simulink model "Diesel_csi"  (R2017a)
settings: Solver=ode4  StartTime=0.0  StopTime=10.0  FixedStep=1e-6  MaxStep=1e-4  RelTol=1e-3
InitFcn:
  | SimulinkInit
values from neighbouring files (symbols this model uses):
  J = 0.3    [SimulinkInit.m]
  K1 = 1.15    [SimulinkInit.m]
  K2 = 1    [SimulinkInit.m]
  K3 = 1    [SimulinkInit.m]
  P = 0.1    [SimulinkInit.m]
  Tao1 = 0.5    [SimulinkInit.m]
  Tao2 = 0.125    [SimulinkInit.m]
undefined symbols (not defined in the file or in its folder): G, GF
libraries: powerlib x16, dsparch4 x3, powerlib_meascontrol x1, simulink x1
settings Model: Creator=Administrador  LastModifiedBy=Administrador
settings OptimizationCC: DefaultParameterBehavior=Inlined  PassReuseOutputArgsAs=Individual arguments
settings DebuggingCC: ParameterTunabilityLossMsg=error
settings SFSimCC: MATLABDynamicMemAlloc=off
settings RTWCC: SystemTargetFile=ert.tlc  TemplateMakefile=ert_default_tmf  Description=Embedded Coder  GenerateReport=on  IncludeHyperlinkInReport=on  LaunchReport=on  GenerateTraceInfo=on  GenerateTraceReport=on  GenerateTraceReportSl=on  GenerateTraceReportSf=on  GenerateTraceReportEml=on
settings CodeAppCC: ForceParamTrailComments=on  IgnoreCustomStorageClasses=off  OperatorAnnotations=on  SimulinkDataObjDesc=on  SFDataObjDesc=on  MATLABFcnDesc=on  InsertBlockDesc=on  MATLABSourceComments=on
settings ERTTargetCC: TargetLangStandard=C99 (ISO)  GenerateSampleERTMain=on  SupportContinuousTime=on  SupportNonInlinedSFcns=on  SupportVariableSizeSignals=on  InlinedParameterPlacement=NonHierarchical  ERTCustomFileTemplate=example_file_process.tlc

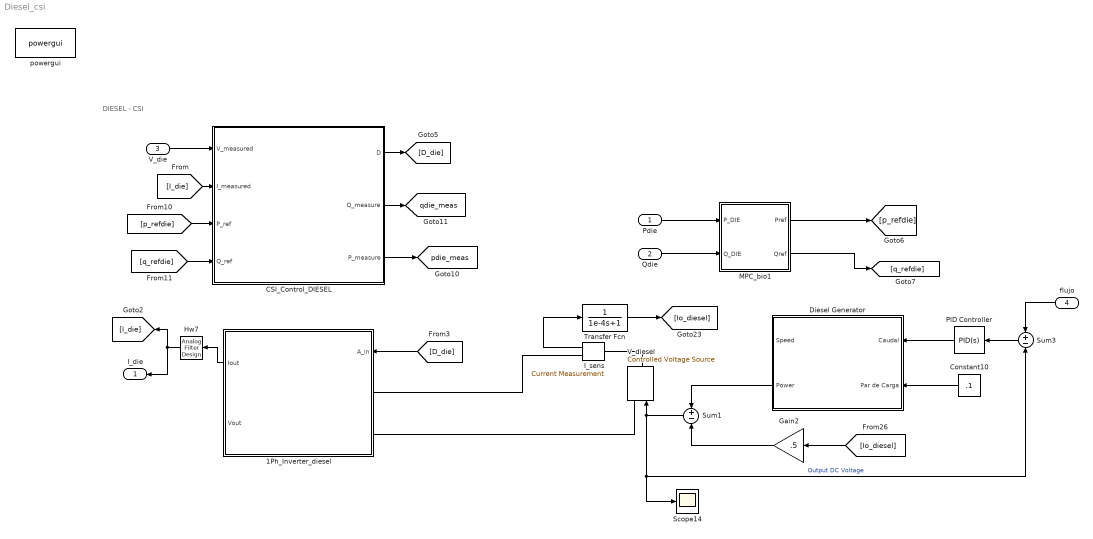
== system Diesel_csi ==
  note: DIESEL - CSI
  Pdie : Inport  PortDimensions=1
  Qdie : Inport  Port=2  PortDimensions=1
  V_die : Inport  Port=3
  flujo : Inport  Port=4
  1Ph_Inverter_diesel : Subsystem  mask{st_time=0, f_sw=12000, samp_f=1e-6}
      mask prompts: st_time "Tiempo muerto (Start)"; f_sw "Switching frequency"; samp_f "Sampling frequency"
      mask Display:
      | port_label('input', 1, 'd', 'texmode', 'on')
      | 
      | port_label('lconn', 1, 'DC +')
      | port_label('lconn', 2, 'DC -')
      | 
      | 
      | port_label('rconn', 1, 'V_{out+}')
      | port_label('rconn', 2, 'B_{out-}')
      | 
      | 
      | port_label('output', 1, 'I_{out}', 'texmode', 'on')
      | port_label('output', 2, 'V_{out}', 'texmode', 'on')
      | 
      | plot([0.1 .9], [0.1 .9])
      | plot([0.2 .4], [.7 .7])
      | plot([0.2 .24], [.65 .65])
      | plot([0.28 .32], [.65 .65])
      | plot([0.36 .40], [.65 .65])
      | 
      | plot([.5:.01:.7], .25+sin(30*[.2:.01:.4])/10)
  CSI_Control_DIESEL : Subsystem  mask{A=[0.0201   -0.039932     0.01986], B=[1     -1.9966       0.998], T=0.0001, st_time=.3, Dn=[1     -1.0364], Dd=[1    -0.96364]}
      mask prompts: A "Numerador del control PR(z)"; B "Denominador del control PR(z)"; T "Tiempo de muestreo"; st_time "Tiempo_muerto"; Dn "Dn (Numerador de D(z))"; Dd "Dd (numerador de D(z))"
      mask DialogControl descripcion Prompt: Lazo de control de corriente para inversor monofasico. La entrada es un setpoint de potencia [P, Q]. Con ese setpoint se calcula la referencia de corriente sinusoidal deacuerdo a la tension medida de la red. Por lo anterior este controlador solo es valido para un inversor conectado a la red pues hara que se comporte como un CSI.
      mask DialogControl Control2 Prompt: Dn y Dd corresponden al numerador y denominador de la funcion de transferencia en Z (denominada D(z)) que hara un desfase de 90 de las señales medidas de tension y corriente del inversor. Estos desfases permiten mimificar las señales alfa y beta, de esta forma usar la misma teoria de potencia instantanea para el caso monofasico.
  Constant10 : Constant  Value=.1
  Diesel Generator : Subsystem
  Gain2 : Gain  Gain=.5
  Hw7 : dsparch4/Analog Filter Design  method=Bessel  filttype=Lowpass  N=2  Wlo=7000*2*pi  Whi=80  Rp=2  Rs=80
  I_sens : powerlib/Measurements/Current Measurement  PhasorSimulation=off  OutputType=Complex  PSBequivalent=0
  MPC_bio1 : Subsystem
  PID Controller : simulink/Continuous/PID Controller  Controller=PID  TimeDomain=Continuous-time  SampleTime=-1  IntegratorMethod=Forward Euler  FilterMethod=Forward Euler  Form=Parallel  UseFilter=on  ControllerParametersSource=internal  P=0.000853612192208084  I=3.94394231511782e-05  D=0.00224356290205903  N=0.155980576752107  InitialConditionSource=internal  InitialConditionForIntegrator=0  InitialConditionForFilter=0  ExternalReset=none  LimitOutput=off  UpperSaturationLimit=inf  LowerSaturationLimit=-inf  LinearizeAsGain=on  AntiWindupMode=none  Kb=1  TrackingMode=off  Kt=1  PParamMin=[]  PParamMax=[]  IParamMin=[]  IParamMax=[]  DParamMin=[]  DParamMax=[]  NParamMin=[]  NParamMax=[]  KbParamMin=[]  KbParamMax=[]  KtParamMin=[]  KtParamMax=[]  POutMin=[]  POutMax=[]  IOutMin=[]  IOutMax=[]  DOutMin=[]  DOutMax=[]  NOutMin=[]  NOutMax=[]  KbOutMin=[]  KbOutMax=[]  KtOutMin=[]  KtOutMax=[]  IntegratorOutMin=[]  IntegratorOutMax=[]  FilterOutMin=[]  FilterOutMax=[]  SumOutMin=[]  SumOutMax=[]  SumI1OutMin=[]  SumI1OutMax=[]  SumI2OutMin=[]  SumI2OutMax=[]  SumI3OutMin=[]  SumI3OutMax=[]  SumDOutMin=[]  SumDOutMax=[]  SaturationOutMin=[]  SaturationOutMax=[]  IntegratorContinuousStateAttributes=''  IntegratorStateMustResolveToSignalObject=off  IntegratorRTWStateStorageClass=Auto  FilterContinuousStateAttributes=''  FilterStateMustResolveToSignalObject=off  FilterRTWStateStorageClass=Auto  DifferentiatorICPrevScaledInput=0  DifferentiatorOutMin=[]  DifferentiatorOutMax=[]  InitialConditionSetting=State (most efficient)
  Scope14 : Scope
  Sum1 : Sum  Inputs=+-
  Sum3 : Sum  Inputs=+-
  Transfer Fcn : TransferFcn  Denominator=[1e-4 1]
  V_diesel : powerlib/Electrical Sources/Controlled Voltage Source  Initialize=on  Source_Type=AC  Amplitude=0  Phase=0  Frequency=0  Measurements=None
  powergui : powerlib/powergui  Priority=1  SimulationMode=Discrete  SampleTime=1e-6  frequency=60  Iterations=50  frequencyindice=0  Pbase=100e6  ErrMax=1e-4  UnitsV=kV  UnitsW=MW  buscounter=0  FunctionMessages=off  echomessages=off  EnableUseOfTLC=off  CurrentSourceSwitches=off  DisableSnubberDevices=off  DisableRonSwitches=off  DisableVfSwitches=off  DisplayEquations=off  SolverType=Tustin/Backward Euler (TBE)  Interpol=off  ExternalGateDelay=off  methode=off  Ts=100  x0status=blocks  SPID=on  SwTol=0  HookPort=off  RestoreLinks=warning  ResistiveCurrentMeasurement=off  Frange=[0:2:500]  Ylog=off  Xlog=on  ShowGrid=off  save=off  variable=ZData  structure=0  ZoomFFT=off  StartTime=0.0  cycles=1  DisplayStyle=1  fundamental=60  FreqAxis=off  MaxFrequency=1000  frequencyindicesteady=1  RmsSteady=1  display=off
  I_die : Outport
  tag scope: pdie_meas=global, qdie_meas=global
  wires:
  [p_refdie] -> CSI_Control_DIESEL/3(P_ref)
  [I_die] -> CSI_Control_DIESEL/2(I_measured)
  CSI_Control_DIESEL/1(D) -> [D_die]
  [D_die] -> 1Ph_Inverter_diesel/1(A_in)
  CSI_Control_DIESEL/2(Q_measure) -> [qdie_meas]
  MPC_bio1/2(Qref) -> [q_refdie]
  Pdie/1 -> MPC_bio1/1(P_DIE)
  1Ph_Inverter_diesel/1(Iout) -> Hw7/1
  Hw7/1 -> I_die/1, [I_die]
  Qdie/1 -> MPC_bio1/2(Q_DIE)
  I_sens/1 -> Transfer Fcn/1
  PID Controller/1 -> Diesel Generator/1(Caudal)
  flujo/1 -> Sum3/1
  Transfer Fcn/1 -> [Io_diesel]
  [Io_diesel] -> Gain2/1
  V_die/1 -> CSI_Control_DIESEL/1(V_measured)
  CSI_Control_DIESEL/3(P_measure) -> [pdie_meas]
  Sum3/1 -> PID Controller/1
  Sum1/1 -> Scope14/1, Sum3/2, V_diesel/1  "Output DC Voltage"
  Constant10/1 -> Diesel Generator/2(Par de Carga)
  MPC_bio1/1(Pref) -> [p_refdie]
  Diesel Generator/2(Power) -> Sum1/1
  Gain2/1 -> Sum1/2
  [q_refdie] -> CSI_Control_DIESEL/4(Q_ref)
  connections:
  I_sens/LConn1 -- V_diesel/RConn1
  I_sens/RConn1 -- 1Ph_Inverter_diesel/LConn1
  V_diesel/LConn1 -- 1Ph_Inverter_diesel/LConn2

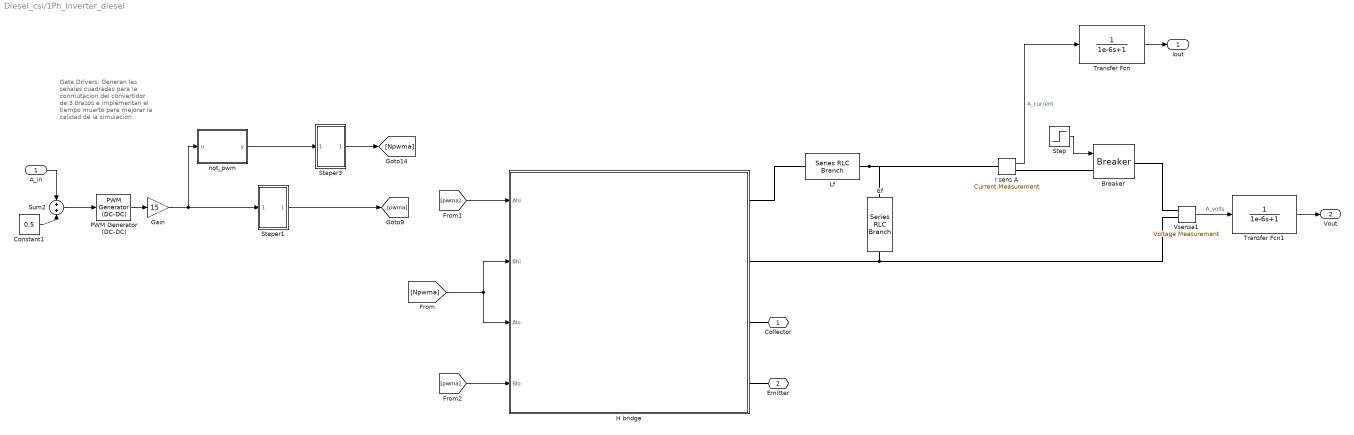
== system Diesel_csi/1Ph_Inverter_diesel ==
  note: Gate Drivers: Generan las señales cuadradas para
      | la conmutacion del convertidor de 3 brazos e implementan el
      | tiempo muerto para mejorar la calidad de la simulacion
  A_in : Inport
  Breaker : powerlib/Elements/Breaker  InitialState=0  SwitchingTimes="[1/60  5/60]"  External=on  BreakerResistance=0.01  SnubberResistance=1e6  SnubberCapacitance=inf  Measurements=None  MoreParameters=on  NoBreakLoop=off
      settings: SourceProductName=Simscape Power Systems
  Cf : powerlib/Elements/Series RLC Branch  LConnTagsString=__new0  RConnTagsString=__new0  BranchType=C  Resistance=1  Inductance=1e-3  SetiL0=off  InitialCurrent=0  Capacitance=22e-6  Setx0=off  InitialVoltage=0  Measurements=None
  Constant1 : Constant  Value=0.5
  Gain : Gain  Gain=15
  H bridge : Subsystem
      mask Display:
      | port_label('input', 1, '\fontsize{12} Ahi', 'texmode', 'on')
      | port_label('input', 2, '\fontsize{12} Alo', 'texmode', 'on')
      | port_label('input', 3, '\fontsize{12} Bhi', 'texmode', 'on')
      | port_label('input', 4, '\fontsize{12} Blo', 'texmode', 'on')
      | 
      | 
      | port_label('rconn', 1, '\fontsize{12} V_{out} +', 'texmode', 'on')
      | port_label('rconn', 2, '\fontsize{12} V_{out} -', 'texmode', 'on')
      | 
      | port_label('rconn', 3, '\fontsize{12} Collector', 'texmode', 'on')
      | port_label('rconn', 4, '\fontsize{12} Emitter', 'texmode', 'on')
      | 
      | lvx = [.1 .1];
      | lvy = [.1 .2];
      | lhx = [.1 .2];
      | lhy = [.1 .1];
      | 
      | 
      | % se dibujan los interruptores de la izquierda
      | plot(lvx+.07, lvy*.8+.028+.1)
      | plot(lvx+.1, lvy+.1)
      | plot(lhx*.5+.15, lhy+.1)
      | plot(lhx*.5+.15, lhy+.2)
      | plot(lhx*.5+.07, lhy+.15)
      | 
      | d=0.5;
      | 
      | plot(lvx+.07, lvy*.8+.028+.1+d)
      | plot(lvx+.1, lvy+.1+d)
      | plot(lhx*.5+.15, lhy+.1+d)
      | plot(lhx*.5+.15, lhy+.2+d)
      | plot(lhx*.5+.07, lhy+.15+d)
      | 
      | 
      | % se dibujan los interruptores del medio
      | h=.3;
      | 
      | %plot(lvx+.07+h, lvy*.8+.028+.1)
      | %plot(lvx+.1+h, lvy+.1)
      | %plot(lhx*.5+.15+h, lhy+.1)
      | %plot(lhx*.5+.15+h, lhy+.2)
      | %plot(lhx*.5+.07+h, lhy+.15)
      | 
      | %plot(lvx+.07+h, lvy*.8+.028+.1+d)
      | %plot(lvx+.1+h, lvy+.1+d)
      | %plot(lhx*.5+.15+h, lhy+.1+d)
      | %plot(lhx*.5+.15+h, lhy+.2+d)
      | %plot(lhx*.5+.07+h, lhy+.15+d)
      | 
      | % se dibujan los interruptores de la derecha
      | h=.6
      | 
      | plot(lvx+.07+h, lvy*.8+.028+.1)
      | plot(lvx+.1+h, lvy+.1)
      | plot(lhx*.5+.15+h, lhy+.1)
      | plot(lhx*.5+.15+h, lhy+.2)
      | plot(lhx*.5+.07+h, lhy+.15)
      | 
      | plot(lvx+.07+h, lvy*.8+.028+.1+d)
      | plot(lvx+.1+h, lvy+.1+d)
      | plot(lhx*.5+.15+h, lhy+.1+d)
      | plot(lhx*.5+.15+h, lhy+.2+d)
      | plot(lhx*.5+.07+h, lhy+.15+d)
      | 
      | 
      | % se conectan los interruptores.
      | plot(lvx+.15, lvy*4-.1)
      | %plot(lvx+.15+.3, lvy*4-.1)
      | plot(lvx+.15+.6, lvy*4-.1)
      | 
      | 
      | plot(lvx+.15, lvy+.7)
      | %plot(lvx+.15+.3, lvy+.7)
      | plot(lvx+.15+.6, lvy+.7)
      | 
      | plot(lvx+.15, lvy)
      | %plot(lvx+.15+.3, lvy)
      | plot(lvx+.15+.6, lvy)
      | 
      | plot(lhx*6-.35, lhy)
      | plot(lhx*6-.35, lhy+.8)
      | 
      | % raul esteban alzate 313 515 86 11
  I sens A : powerlib/Measurements/Current Measurement  PhasorSimulation=off  OutputType=Complex  PSBequivalent=0
  Lf : powerlib/Elements/Series RLC Branch  LConnTagsString=__new0  RConnTagsString=__new0  BranchType=RL  Resistance=.1  Inductance=30e-3  SetiL0=off  InitialCurrent=0  Capacitance=1e-6  Setx0=off  InitialVoltage=0  Measurements=None
  PWM Generator (DC-DC) : powerlib_meascontrol/Pulse & Signal Generators/PWM Generator (DC-DC)  Fsw=f_sw  Ts=samp_f
  Step : Step  Time=st_time  SampleTime=0
  Steper1 : Subsystem
  Steper3 : Subsystem
  Sum2 : Sum
  Transfer Fcn : TransferFcn  Denominator=[1e-6 1]
  Transfer Fcn1 : TransferFcn  Denominator=[1e-6 1]
  Vsensa1 : powerlib/Measurements/Voltage Measurement  PhasorSimulation=off  OutputType=Complex  PSBequivalent=0
  not_pwm : MATLAB Function  TreatAsAtomicUnit=on
  Collector : PMIOPort  Port=1  Side=Left
  Emitter : PMIOPort  Port=2  Side=Left
  Iout : Outport
  Vout : Outport  Port=2
  wires:
  Vsensa1/1 -> Transfer Fcn1/1  "A_volts"
  I sens A/1 -> Transfer Fcn/1  "A_current"
  [pwma] -> H bridge/4(Blo)
  [Npwma] -> H bridge/3(Alo), H bridge/2(Bhi)
  [pwma] -> H bridge/1(Ahi)
  Gain/1 -> not_pwm/1(u), Steper1/1(In1)
  Steper3/1(Out1) -> [Npwma]
  Steper1/1(Out1) -> [pwma]
  A_in/1 -> Sum2/1
  Constant1/1 -> Sum2/2
  PWM Generator (DC-DC)/1 -> Gain/1
  Sum2/1 -> PWM Generator (DC-DC)/1
  not_pwm/1(y) -> Steper3/1(In1)
  Transfer Fcn/1 -> Iout/1
  Transfer Fcn1/1 -> Vout/1
  Step/1 -> Breaker/1
  connections:
  Cf/RConn1 -- Vsensa1/LConn2 -- H bridge/RConn2
  Lf/LConn1 -- H bridge/RConn1
  H bridge/RConn4 -- Emitter/RConn1
  H bridge/RConn3 -- Collector/RConn1
  Breaker/LConn1 -- I sens A/RConn1
  Vsensa1/LConn1 -- Breaker/RConn1
  Lf/RConn1 -- I sens A/LConn1 -- Cf/LConn1

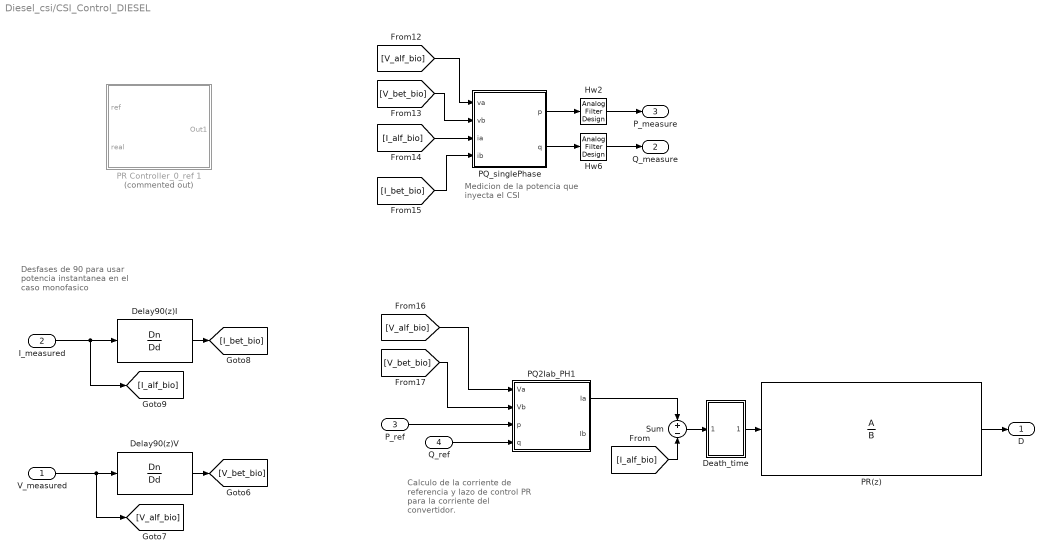
== system Diesel_csi/CSI_Control_DIESEL ==
  note: Calculo de la corriente de referencia
      | y lazo de control PR para la corriente
      | del convertidor.
  note: Desfases de 90 para usar potencia
      | instantanea en el caso monofasico
  note: Medicion de la potencia que inyecta el CSI
  V_measured : Inport
  I_measured : Inport  Port=2
  P_ref : Inport  Port=3
  Q_ref : Inport  Port=4
  Death_time : Subsystem
  Delay90(z)I : DiscreteTransferFcn  Numerator=Dn  Denominator=Dd  SampleTime=T
  Delay90(z)V : DiscreteTransferFcn  Numerator=Dn  Denominator=Dd  SampleTime=T
  Hw2 : dsparch4/Analog Filter Design  method=Bessel  filttype=Lowpass  N=4  Wlo=30*2*pi  Whi=80  Rp=2  Rs=80
  Hw6 : dsparch4/Analog Filter Design  method=Bessel  filttype=Lowpass  N=4  Wlo=30*2*pi  Whi=80  Rp=2  Rs=80
  PQ2Iab_PH1 : MATLAB Function  TreatAsAtomicUnit=on
  PQ_singlePhase : MATLAB Function  TreatAsAtomicUnit=on
  PR Controller_0_ref 1 : Subsystem  Commented=on  mask{Kp=40/100, Ki=200, wa=2, w0=60*2*pi, st_time=1e-3}
      mask prompts: Kp "Ganancia Proporcional"; Ki "Ganancia Integral"; wa "Ancho camapana resonancia"; w0 "Frecuencia Central"; st_time "Tiempo muerto (Start)"
      mask Display:
      | port_label('input',1,'ref')
      | port_label('input',2,'sens')
      | port_label('output',1,'out')
      | 
      | plot(.4+[0:.01:pi/10], .32+sin(40*[0:.01:pi/10])/13)
      | 
      | plot([.4 .6],.05+[.5 .7])
      | plot([.4 .6],.05+[.9 .7])
      | plot([.4 .4],.05+[.9 .5])
      | 
      | text(.27,.37,'\fontsize{25} \int', 'texmode', 'on')
  PR(z) : DiscreteTransferFcn  Numerator=A  Denominator=B  SampleTime=T
  Sum : Sum  Inputs=+-
  D : Outport
  Q_measure : Outport  Port=2
  P_measure : Outport  Port=3
  wires:
  PR(z)/1 -> D/1
  Sum/1 -> Death_time/1(In1)
  PQ2Iab_PH1/1(Ia) -> Sum/1
  [I_alf_bio] -> Sum/2
  Death_time/1(Out1) -> PR(z)/1
  Q_ref/1 -> PQ2Iab_PH1/4(q)
  P_ref/1 -> PQ2Iab_PH1/3(p)
  PQ_singlePhase/2(q) -> Hw6/1
  V_measured/1 -> [V_alf_bio], Delay90(z)V/1
  [V_alf_bio] -> PQ_singlePhase/1(va)
  [V_bet_bio] -> PQ_singlePhase/2(vb)
  Delay90(z)V/1 -> [V_bet_bio]
  Hw2/1 -> P_measure/1
  [V_alf_bio] -> PQ2Iab_PH1/1(Va)
  [I_alf_bio] -> PQ_singlePhase/3(ia)
  [I_bet_bio] -> PQ_singlePhase/4(ib)
  Delay90(z)I/1 -> [I_bet_bio]
  [V_bet_bio] -> PQ2Iab_PH1/2(Vb)
  Hw6/1 -> Q_measure/1
  PQ_singlePhase/1(p) -> Hw2/1
  I_measured/1 -> [I_alf_bio], Delay90(z)I/1

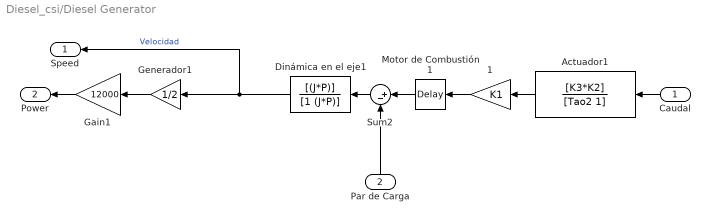
== system Diesel_csi/Diesel Generator ==
  Caudal : Inport
  Par de Carga : Inport  Port=2
  " 1" : Gain  Gain=K1
  " Generador1" : Gain  Gain=1/2
  Actuador1 : TransferFcn  Numerator=[K3*K2]  Denominator=[Tao2 1]
  Dinámica en el eje1 : TransferFcn  Numerator=[(J*P)]  Denominator=[1 (J*P)]
  Gain1 : Gain  Gain=12000
  Motor de Combustión1 : TransportDelay  DelayTime=Tao1
  Sum2 : Sum  Inputs=|+-
  Speed : Outport
  Power : Outport  Port=2
  wires:
  " 1"/1 -> Motor de Combustión1/1
  " Generador1"/1 -> Gain1/1
  Motor de Combustión1/1 -> Sum2/1
  Actuador1/1 -> " 1"/1
  Dinámica en el eje1/1 -> Speed/1, " Generador1"/1  "Velocidad"
  Sum2/1 -> Dinámica en el eje1/1
  Caudal/1 -> Actuador1/1
  Par de Carga/1 -> Sum2/2
  Gain1/1 -> Power/1

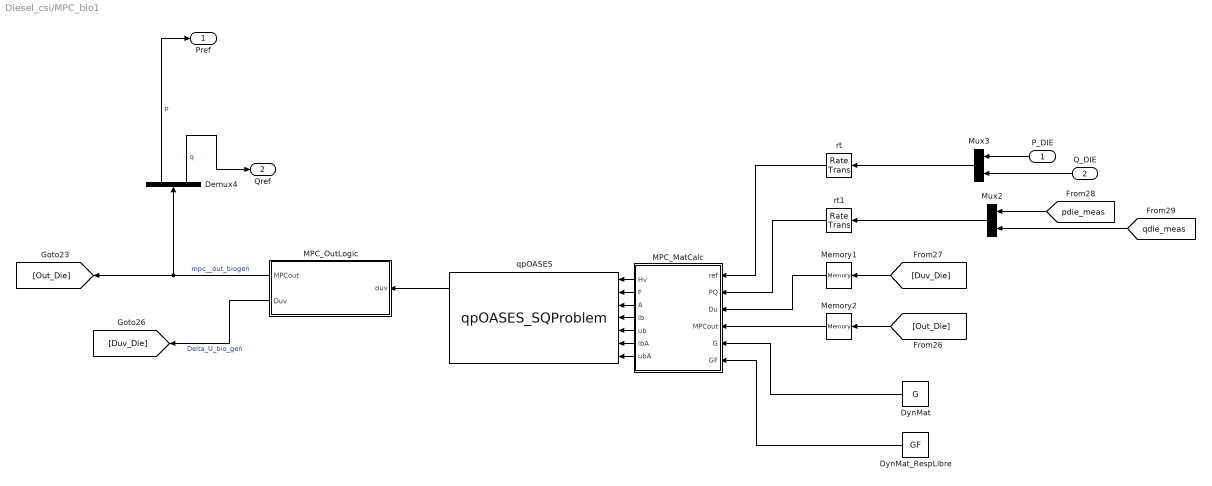
== system Diesel_csi/MPC_bio1 ==
  P_DIE : Inport
  Q_DIE : Inport  Port=2
  Demux4 : Demux  Outputs=2
  DynMat : Constant  Value=G
  DynMat_RespLibre : Constant  Value=GF
  MPC_MatCalc : MATLAB Function  TreatAsAtomicUnit=on  SystemSampleTime=1e-3
      settings: MinAlgLoopOccurrences=on
  MPC_OutLogic : MATLAB Function  TreatAsAtomicUnit=on
      settings: MinAlgLoopOccurrences=on
  Memory1 : Memory
  Memory2 : Memory
  Mux2 : Mux  Inputs=2
  Mux3 : Mux  Inputs=2
  qpOASES : S-Function  FunctionName=qpOASES_SQProblem  SFunctionDeploymentMode=off  EnableBusSupport=off
  rt : RateTransition  X0=[0 0]  OutPortSampleTime=1e-3
  rt1 : RateTransition  X0=[0 0]  OutPortSampleTime=1e-3
  Pref : Outport
  Qref : Outport  Port=2
  wires:
  [Out_Die] -> Memory2/1
  MPC_MatCalc/7(ubA) -> qpOASES/7
  MPC_MatCalc/6(lbA) -> qpOASES/6
  MPC_MatCalc/2(F) -> qpOASES/2
  rt1/1 -> MPC_MatCalc/2(PQ)
  Memory1/1 -> MPC_MatCalc/3(Du)
  [Duv_Die] -> Memory1/1
  MPC_MatCalc/5(ub) -> qpOASES/5
  MPC_OutLogic/1(MPCout) -> [Out_Die], Demux4/1  "mpc__out_biogen"
  DynMat_RespLibre/1 -> MPC_MatCalc/6(GF)
  DynMat/1 -> MPC_MatCalc/5(G)
  Demux4/1 -> Pref/1  "p"
  Memory2/1 -> MPC_MatCalc/4(MPCout)
  MPC_MatCalc/3(A) -> qpOASES/3
  MPC_MatCalc/1(Hv) -> qpOASES/1
  MPC_OutLogic/2(Duv) -> [Duv_Die]  "Delta_U_bio_gen"
  MPC_MatCalc/4(lb) -> qpOASES/4
  rt/1 -> MPC_MatCalc/1(ref)
  qpOASES/1 -> MPC_OutLogic/1(duv)
  Mux2/1 -> rt1/1
  Mux3/1 -> rt/1
  [pdie_meas] -> Mux2/1
  Q_DIE/1 -> Mux3/2
  [qdie_meas] -> Mux2/2
  Demux4/2 -> Qref/1  "q"
  P_DIE/1 -> Mux3/1

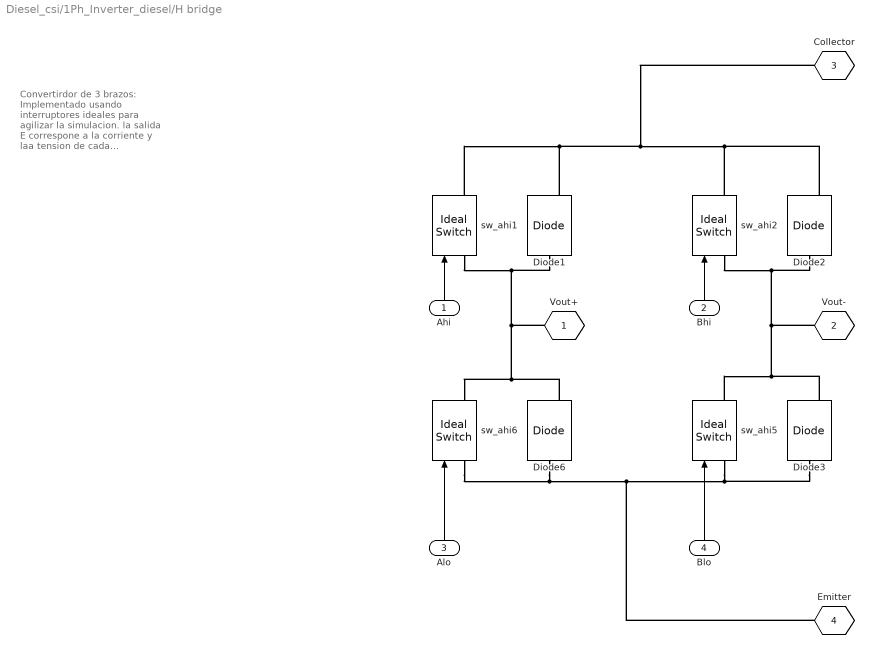
== system Diesel_csi/1Ph_Inverter_diesel/H bridge ==
  note: Convertirdor de 3 brazos:
      |
      | Implementado usando interruptores
      | ideales para agilizar la simulacion.
      | la salida E correspone a la corriente y laa
      | tension de cada componente
      | (sea interruptor o diodo) y su respectiva
      | corriente. no tienen puerto de salida ya que no
      | son relevantes para lo que se desea simular.
      |
      | si g=0 interruptor no conduce.
      | si g=1 interruptor conduce.
      |
      | conmutacion ocurre instantaneamente sin
      | retardo.
  Ahi : Inport
  Bhi : Inport  Port=2
  Alo : Inport  Port=3
  Blo : Inport  Port=4
   sw_ahi{1..2,5..6} (4 alike) : powerlib/Power Electronics/Ideal Switch  Ron=0.1  Lon=0  IC=0  Rs=1e6  Cs=10e-12  Measurements=on
  Diode{1..3,6} (4 alike) : powerlib/Power Electronics/Diode  Ron=.2  Lon=0  Vf=0.8  IC=0  UseSnubber=0  Rs=0  Cs=0  Measurements=on
  " Vout+" : PMIOPort  Tag=PMCPort  Port=1  Side=Right
  Vout- : PMIOPort  Tag=PMCPort  Port=2  Side=Right
  Collector : PMIOPort  Tag=PMCPort  Port=3  Side=Right
  Emitter : PMIOPort  Tag=PMCPort  Port=4  Side=Right
  wires:
  Bhi/1 -> " sw_ahi2"/1
  Blo/1 -> " sw_ahi5"/1
  Ahi/1 -> " sw_ahi1"/1
  Alo/1 -> " sw_ahi6"/1
  connections:
  " sw_ahi1"/LConn1 -- Diode1/LConn1 -- " Vout+"/RConn1 -- Diode6/RConn1 -- " sw_ahi6"/RConn1
  " sw_ahi2"/RConn1 -- Diode1/RConn1 -- " sw_ahi1"/RConn1 -- Collector/RConn1 -- Diode2/RConn1
  " sw_ahi5"/LConn1 -- " sw_ahi6"/LConn1 -- Diode6/LConn1 -- Emitter/RConn1 -- Diode3/LConn1
  " sw_ahi5"/RConn1 -- Diode2/LConn1 -- " sw_ahi2"/LConn1 -- Vout-/RConn1 -- Diode3/RConn1

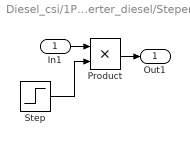
== system Diesel_csi/1Ph_Inverter_diesel/Steper1 ==
  In1 : Inport
  Product : Product
  Step : Step  Time=st_time  SampleTime=samp_f
  Out1 : Outport
  wires:
  Product/1 -> Out1/1
  In1/1 -> Product/1
  Step/1 -> Product/2

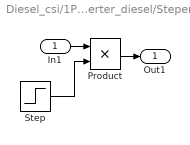
== system Diesel_csi/1Ph_Inverter_diesel/Steper3 ==
  In1 : Inport
  Product : Product
  Step : Step  Time=st_time  SampleTime=samp_f
  Out1 : Outport
  wires:
  Step/1 -> Product/2
  In1/1 -> Product/1
  Product/1 -> Out1/1

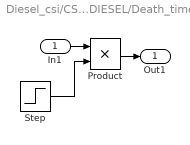
== system Diesel_csi/CSI_Control_DIESEL/Death_time ==
  In1 : Inport
  Product : Product
  Step : Step  Time=st_time  SampleTime=T
  Out1 : Outport
  wires:
  Step/1 -> Product/2
  In1/1 -> Product/1
  Product/1 -> Out1/1

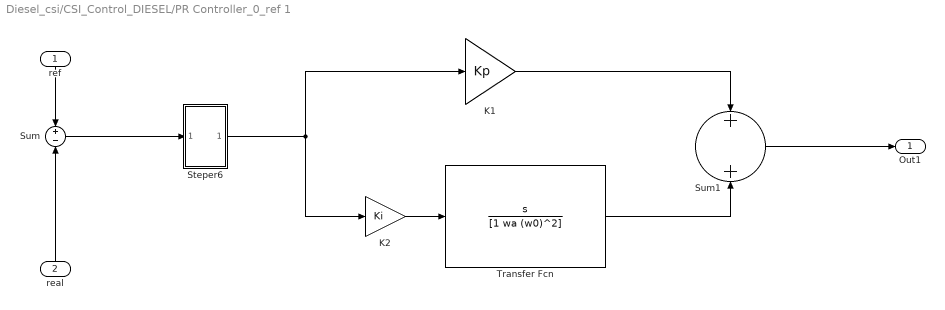
== system Diesel_csi/CSI_Control_DIESEL/PR Controller_0_ref 1 ==
  ref : Inport
  real : Inport  Port=2
  K1 : Gain  Gain=Kp
  K2 : Gain  Gain=Ki
  Steper6 : Subsystem
  Sum : Sum  Inputs=+-
  Sum1 : Sum  Inputs=+|+
  Transfer Fcn : TransferFcn  Numerator=[1 0]  Denominator=[1 wa (w0)^2]
  Out1 : Outport
  wires:
  Sum1/1 -> Out1/1
  Steper6/1(Out1) -> K2/1, K1/1
  K2/1 -> Transfer Fcn/1
  Transfer Fcn/1 -> Sum1/2
  K1/1 -> Sum1/1
  Sum/1 -> Steper6/1(In1)
  ref/1 -> Sum/1
  real/1 -> Sum/2

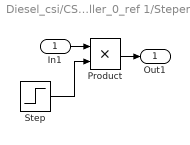
== system Diesel_csi/CSI_Control_DIESEL/PR Controller_0_ref 1/Steper6 ==
  In1 : Inport
  Product : Product
  Step : Step  Time=st_time  SampleTime=0
  Out1 : Outport
  wires:
  Step/1 -> Product/2
  In1/1 -> Product/1
  Product/1 -> Out1/1

== matlab function Diesel_csi/1Ph_Inverter_diesel/not_pwm ==
  data: u input; y output
function y = fcn(u)
%#codegen

if(u==0 || u<0)
    a=15;
else
    a=0;
end;

y = a;

== matlab function Diesel_csi/CSI_Control_DIESEL/PQ2Iab_PH1 ==
  data: Va input; Ia output; Vb input; p input; q input; Ib output
function [Ia, Ib] = fcn(Va, Vb, p, q)
%#codegen

% divide by zero protection
if(abs((Va^2+Vb^2))<=1000*eps(0))
    det = 1/eps(0);
else
    det = 1/(Va^2+Vb^2); % constante auxiliar
end;
%det = 1/(Va^2+Vb^2);

Mat = det*[Va Vb; Vb -Va];
Iab = Mat*[2*p;2*q];

Iaaux = Iab(1);
Ibaux = Iab(2);

ilim=1e3;

if(Iaaux>ilim)
    Iaaux=ilim;
end;
if(Iaaux<-ilim)
    Iaaux =-ilim;    
end;

if(isnan(Iaaux))
    Iaaux=0;
end;
%-----------------


if(Ibaux>ilim)
    Ibaux=ilim;
end;
if(Ibaux<-ilim)
    Ibaux =-ilim;    
end;

if(isnan(Ibaux))
    Ibaux=0;
end;
%-----------------


Ia = Iaaux;
Ib = Ibaux;

== matlab function Diesel_csi/CSI_Control_DIESEL/PQ_singlePhase ==
  data: va input; p output; vb input; ia input; ib input; q output
function [p, q] = fcn(va, vb, ia, ib)
% Esta funcion calcula la potencia activa y reactiva instantanea
% para el caso mnosofasico. En la revision de 2 papers he observado
% que una manera de extender la teoria de potencia al caso monofasico
% es asumiendo la tension o corriente de una fase como la componente
% alpha y hacer un desfase de 90 grados para obtener una version
% artificial de beta.

paux=va*ia+vb*ib;
if(paux > 20e4)
    paux = 20e4;
end
if(paux < -20e4)
    paux = -20e-4;
end

p = paux/2; % potencia activa instantanea

qaux = vb*ia-va*ib;

if(qaux>20e4)
    qaux=20e4;
end
if(qaux<-20e4)
    qaux=-20e4;
end

q = qaux/2; % potencia reactiva instantanea

== matlab function Diesel_csi/MPC_bio1/MPC_MatCalc ==
  data: ref input; PQ input; Hv output; F output; A output; lb output; ub output; lbA output; ubA output; Du input; MPCout input; G input; GF input
function [Hv, F, A, lb, ub, lbA, ubA] = MPC(ref, PQ, Du, MPCout, G, GF)

%%parametros del MPC


p = 100; % horizonte de prediccion
Nu = 100; % horizonte de control


%% Calculo de la salida de control.

H = G'*G+eye(2*Nu)*3000; % parte cuadratica del qp

ym = [ ones(p, 1)*PQ(1); ones(p, 1)*PQ(2) ]; % vector de la medida de tempearatura actual.

w = [ ones(p, 1)*ref(1); ones(p, 1)*ref(2) ]; % vector señal setpoint.

L = GF*Du+ym; % respuesta libre.

F = 2*(L-w)'*G; % parte lineal del problema qp.

A = zeros(1, 4*Nu*Nu);

lbA = zeros(1, 2*Nu);

ubA = zeros(1, 2*Nu);

Hv = M2V(H);

hip = HiBound(MPCout(1), 600, 10);
hiq = HiBound(MPCout(2), 5000, 1000);

lop = LowBound(MPCout(1), -100, -10);
loq = LowBound(MPCout(2), -100, -1000);

lb = [ones(1, Nu)*lop ones(1, Nu)*loq];
ub = [ones(1, Nu)*hip ones(1, Nu)*hiq];
end

% el control mpc implementado halla mediante programacion cuadratica
% los delta de u optimos deacuerdo a la funcion de coste. por este motivo
% es necesario implementar una logica adicional que permita limitar
% los valores de u (la salida) ya que estos no se manupilan directamente
% en el problema de programacion cuadratica.

% esta logica se implementan en las dos funciones locales que se encuentran
% a continuacion. una funcion define el limite superior y otra funcion para
% definir el limite inferior de los deltas de u deacuerdo al valor actual
% de u para asegurar que tanto los deltas de u como el valor de u esten
% limitados.
% esta funcion solo es correcta si max y Dmax son valores positivos.
function y = HiBound(X, max, Dmax)
    if(X>=0) % si la potencia X es positiva:
        if(max >= X)% si X no ha superado la potencia maxima:
            if(max-X >= Dmax) % si la distancia supera el cambio maximo deseado
                r = Dmax;
            else % si es menor al cambio maximo deseado
                r = max-X;
            end
        else % si X supera la potencia maxima deseada
            r = 0; % el delta maximo es 0 para que no se incremente mas.
        end
    else % si la potencia X es negativa, el incremento maximo es
        r = Dmax;
    end
    y = r;
end

% esta funcion para el lower bound se penso para trbajar con valores
% negativos. si min y Dmin no es negativo la funcion no funciona
% correctamente.
function y = LowBound(X, minv, Dmin)
    if(X<=0) % si la potencia X esta en el cuadrante inferior:
        if(minv <= X)% si X es mayor que la potencia minima:
            if(minv-X <= Dmin) % si la distancia supera el cambio maximo deseado
                r = Dmin;
            else % si es mayor al cambio maximo deseado
                r = minv-X;
            end
        else % si X es menor la potencia maxima deseada
            r = 0; % el delta maximo es 0 para que no se decremente mas.
        end
    else % si la potencia X es positiva, el decremento maximo es
        r = Dmin;
    end
    y = r;
end

== matlab function Diesel_csi/MPC_bio1/MPC_OutLogic ==
  data: MPCout output; duv input; Duv output
function [MPCout, Duv] = MPC_out_Logic(duv)

%%parametros del MPC
Nu = 100; % horizonte de control.


%% variables del MPC
persistent Du; % deltas de u 
persistent out; % salida actual del conrolador MPC.

if isempty(Du) % inicializacion de los deltas de uu
    Du = zeros(2*Nu, 1);
end

if isempty(out) % inicializaion de la salida del controlador MPC
    out = [0; 0];
end


du = [duv(1), duv(Nu+1)];


Du = [du(1); Du(1:Nu-1); du(2); Du(Nu+1:end-1)];% actualizar historial deltas de u.

out = [ out(1)+du(1); out(2)+du(2) ]; %calcular salida del controlador.

MPCout = out;
Duv = Du;
